simulink library "CPC5_SFUN_wrapper"  (Simulink 8.7)
settings: Solver=VariableStepAuto  SolverMode=SingleTasking  StartTime=0.0  StopTime=10.0  RelTol=1e-3
PreLoadFcn:
  | CPC5_SFUN_PreLoadFcn
  | CPC5_SFUN_InitFcn
undefined symbols (not defined in the file): user_config
settings Model: Creator=Silver T-2022.03-4  LastModifiedBy=pjhaver

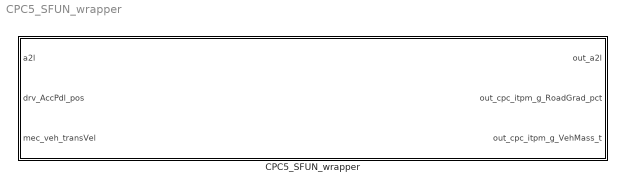
== system CPC5_SFUN_wrapper ==
  CPC5_SFUN_wrapper : Subsystem
      mask Display:
      | patch(.5 + 0.03*8*cos(0:pi/50:2*pi),   .5 + 0.14675 *8*sin(0:pi/50:2*pi), [0 0 1])
      | patch(.5 + 0.03*[6.5, 8, 0, -1.5],     .5 + 0.14675 *[-8,-6.5, 1.5, 0], [.8, .8, .8])
      | patch(.5 + 0.03*5.5*cos(0:pi/50:2*pi), .5 + 0.14675 *5.5*sin(0:pi/50:2*pi), [.8, .8, .8])
      | patch(.5 + 0.03*3.5*cos(0:pi/50:2*pi), .5 + 0.14675 *3.5*sin(0:pi/50:2*pi), [0 0 1])

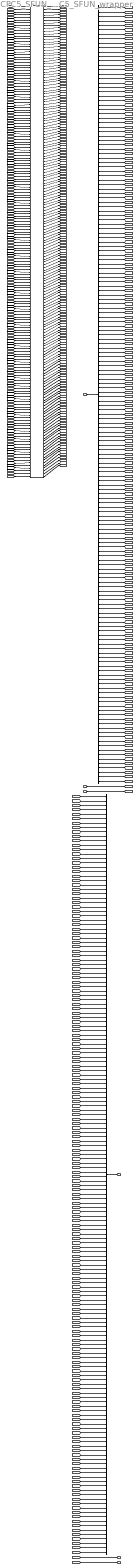
== system CPC5_SFUN_wrapper/CPC5_SFUN_wrapper ==
  a2l : Inport  OutDataTypeStr=Bus:a2l_1
  drv_AccPdl_pos : Inport  Port=2
  mec_veh_transVel : Inport  Port=3
  BusCreator183 : BusCreator  Inputs=172
  BusSelector1 : BusSelector  OutputSignals=ch_Accel_X_Cval,ch_AirTempOutsd_Cval_SCA,ch_AutoManSw_Rq_SAM,ch_BS_Brk_Cval,ch_BS_CSCPC_Acc_Stat,ch_BS_CSCPC_Intf_Stat,ch_BS_CSCPC_RqPerf_Stat,ch_BS_HB_RqPerf_Stat,ch_BrkPdlPosn3_Cval,ch_CC_DecHystSw_Rq,ch_CC_DecLoHystSw_Rq,ch_CC_HystSpd_Rq_ICUC,ch_CC_IncHystSw_Rq,ch_CC_IncLoHystSw_Rq,ch_CC_LowHystSpd_Rq_ICUC,ch_CstValIPPC_Rq,ch_CurvSpd_Rq,ch_DateTmDay_Cval_ICUC,ch_DateTmHour_Cval_ICUC,ch_DateTmMinute_Cval_ICUC,ch_DateTmMonth_Cval_ICUC,ch_DateTmSecond_Cval_ICUC,ch_DateTmYear_Cval_ICUC,ch_DiffLkIAC_Stat,ch_DipHystSpd_Rq,ch_DrvMdSwNorm_Rq_SAM,ch_EBS_BrkSw2_Rq,ch_EngRetTrqMax_Rq,ch_EngRetTrqMin_Rq,ch_GrSelSw_Rq_SAM,ch_HillHolderAvl_Stat,ch_IgnSw_Stat_SCA,ch_RetSwPos_Rq_SAM,ch_RoadCurv_Cval,ch_SFA_Ind_Stat,ch_SelSpdUnit_Stat,ch_SpdFtAxleLtWhl_Cval,ch_SpdFtAxleRtWhl_Cval,ch_SpdR_AxleLtWhl_Cval,ch_SpdR_AxleRtWhl_Cval,ch_SrcAdrBrkCtrlDev_Cval,ch_StW_Sw09_Rq,ch_StW_Sw10_Rq,ch_StW_Sw11_Rq,ch_StW_Sw13_Rq,ch_TotalVehDist_Cval_DIAG,ch_TrfGrBoxRng_Stat,ch_TyreRollCircumFA_Cval,ch_TyreRollCircumRA_Cval,ch_VehMtnDet_Stat_ICUC,ch_XBR_AccelLim_Stat_BS,pt_AbsMaxEngTrq_Cval_PT,pt_AbsMaxRetTrq_Cval_PT,pt_ActlMaxEngSpd_Cval_PT,pt_ActlMaxRetTrqNoTemp_Cval,pt_BoostPress_Cval_PT,pt_CC_MdDem_Rq,pt_Clutch_Cval_PT,pt_Clutch_Stat_TCM_PT,pt_CoolTempIn_Cval_PT,pt_CoolTempOut_Cval_PT,pt_CoolTempRet_Cval_PT,pt_CoolTemp_Cval_PT,pt_CreepAct_Stat_PT,pt_CreepMaxTrq_Cval_PT,pt_CurrGr_Stat_PT,pt_DeclSens_Cval_PT,pt_DrvDirByGr_Stat_TCM_PT,pt_DrvDirec_Stat_TCM_PT,pt_DrvlineEngg_Stat_PT,pt_EbmReq_IPPC,pt_EcoMode_Rq_PPC,pt_EngBrk1_Stat_MR_PT,pt_EngBrk2_Stat_MR_PT,pt_EngFrictTrq_Cval_PT,pt_EngHours_Cval_PT,pt_EngIdleSpd_Cval_MCM_PT,pt_EngIdleSpd_Rq_TCM_PT,pt_EngIdle_Stat_MCM,pt_EngIgn_Stat_MCM,pt_EngMode_Stat_MCM,pt_EngSpd_Cval_PT,pt_EngSpd_Rq_TCM_PT,pt_EngStSpInhbt_Rq_MCM,pt_EngTrqDecRate_Cval_PT,pt_EngTrq_Cval_PT,pt_FEL_Rq_IPPC,pt_FanSpdPct_Cval_PT,pt_FanSpd_Cval_PT,pt_FuelCons_Cval_PT,pt_FuelMapEngSpd_Cval_PT,pt_FuelMapNum_Cval_PT,pt_FuelMapSelNum_Cval_PT,pt_FuelMapTrqNoBst_Cval_PT,pt_FwdGr10_Stat_PT,pt_FwdGr11_Stat_PT,pt_FwdGr12_Stat_PT,pt_FwdGr13_Stat_PT,pt_FwdGr14_Stat_PT,pt_FwdGr15_Stat_PT,pt_FwdGr16_Stat_PT,pt_FwdGr1_Stat_PT,pt_FwdGr2_Stat_PT,pt_FwdGr3_Stat_PT,pt_FwdGr4_Stat_PT,pt_FwdGr5_Stat_PT,pt_FwdGr6_Stat_PT,pt_FwdGr7_Stat_PT,pt_FwdGr8_Stat_PT,pt_FwdGr9_Stat_PT,pt_GrShift_Stat_PT,pt_HystSpd_Cval_IPPC,pt_IPPC_Stat,pt_InShaftSpd_Cval_PT,pt_IntrUrbUcReq_IPPC,pt_LoHystSpd_Cval_IPPC,pt_LowSpd_Cval_IPPC,pt_MapRoadGrad_Cval,pt_MaxAccel_Rq_IPPC,pt_MaxActlEngTrq_Cval_PT,pt_MaxEngBrk_Rq_IPPC,pt_MaxEngTrq_Rq_PT,pt_MaxRetTrq_Cval_PT,pt_MinAccel_Rq_IPPC,pt_MinEngBrk_Rq_IPPC,pt_MinEngTrq_Rq_PT,pt_MinRetTrqPwrUp_Stat_PT,pt_NeuRangeGroup_Stat_PT,pt_NeuRangeHigh_Stat_PT,pt_NeuRangeLow_Stat_PT,pt_NeuSplitGroup_Stat_PT,pt_NeuSplitHigh_Stat_PT,pt_NeuSplitLow_Stat_PT,pt_OutShaftSpd_Cval_PT,pt_PThM_Blind_Rq_PT,pt_PThM_FanCtrl_Rq,pt_PThM_WtrPmp_Rq_PT,pt_PthM_ThstHeat_Rq_PT,pt_ReqTrq_Cval_IPPC,pt_RetActv_Stat_PT,pt_RetOilTemp_Cval_PT,pt_RetTrqMd_Stat,pt_RetTrq_Cval_PT,pt_RevGr2_Stat_PT,pt_RevGr3_Stat_PT,pt_RevGr4_Stat_PT,pt_RotSens_Stat_PT,pt_SOC_Range_Rq_IPPC,pt_SaveSetSpd_Rq_IPPC,pt_SelGr_Rq_IPPC,pt_SelGr_Stat_PT,pt_SelSpdController_Rq_PT,pt_SetSpd_Cval_IPPC,pt_ShiftSprtEng_Rq_TCM,pt_ShiftTimeDown1_Cval_PT,pt_ShiftTimeDown2_Cval_PT,pt_ShiftTimeDown3_Cval_PT,pt_ShiftTimeDown4_Cval_PT,pt_ShiftTimeUp1_Cval_PT,pt_ShiftTimeUp2_Cval_PT,pt_ShiftTimeUp3_Cval_PT,pt_ShiftTimeUp4_Cval_PT,pt_SysID_CCM,pt_SysID_MCM,pt_SysID_RCM,pt_SysID_TCM,pt_ThermoRoll_Rq,pt_TopTrq_Rq_IPPC,pt_TrqConvLkup_Stat_PT,pt_TrqConv_Cval_PT,pt_TrqConv_Stat_PT,pt_TxActlGrRatio_Cval_PT,pt_UpSpd_Cval_IPPC,pt_UseCase_Rq_IPPC,pt_XBR_Rq_IPPC,drv_ign
  sfunction : S-Function  FunctionName=CPC5_SFUN  Parameters=user_config  SFunctionDeploymentMode=off  EnableBusSupport=off  mask{user_config=user_config}
  out_a2l : Outport
  out_cpc_itpm_g_RoadGrad_pct : Outport  Port=2
  out_cpc_itpm_g_VehMass_t : Outport  Port=3
  wires:
  [L2] -> sfunction/1
  [L3] -> sfunction/2
  [L4] -> sfunction/3
  [L5] -> sfunction/4
  [L6] -> sfunction/5
  [L7] -> sfunction/6
  [L8] -> sfunction/7
  [L9] -> sfunction/8
  [L10] -> sfunction/9
  [L11] -> sfunction/10
  [L12] -> sfunction/11
  [L13] -> sfunction/12
  [L14] -> sfunction/13
  [L15] -> sfunction/14
  [L16] -> sfunction/15
  [L17] -> sfunction/16
  [L18] -> sfunction/17
  [L19] -> sfunction/18
  [L20] -> sfunction/19
  [L21] -> sfunction/20
  [L22] -> sfunction/21
  [L23] -> sfunction/22
  [L24] -> sfunction/23
  [L25] -> sfunction/24
  [L26] -> sfunction/25
  [L27] -> sfunction/26
  [L28] -> sfunction/27
  [L29] -> sfunction/28
  [L30] -> sfunction/29
  [L31] -> sfunction/30
  [L32] -> sfunction/31
  [L33] -> sfunction/32
  [L34] -> sfunction/33
  [L35] -> sfunction/34
  [L36] -> sfunction/35
  [L37] -> sfunction/36
  [L38] -> sfunction/37
  [L39] -> sfunction/38
  [L40] -> sfunction/39
  [L41] -> sfunction/40
  [L42] -> sfunction/41
  [L43] -> sfunction/42
  [L44] -> sfunction/43
  [L45] -> sfunction/44
  [L46] -> sfunction/45
  [L47] -> sfunction/46
  [L48] -> sfunction/47
  [L49] -> sfunction/48
  [L50] -> sfunction/49
  [L51] -> sfunction/50
  [L52] -> sfunction/51
  [L53] -> sfunction/52
  [L54] -> sfunction/53
  [L55] -> sfunction/54
  [L56] -> sfunction/55
  [L57] -> sfunction/56
  [L58] -> sfunction/57
  [L59] -> sfunction/58
  [L60] -> sfunction/59
  [L61] -> sfunction/60
  [L62] -> sfunction/61
  [L63] -> sfunction/62
  [L64] -> sfunction/63
  [L65] -> sfunction/64
  [L66] -> sfunction/65
  [L67] -> sfunction/66
  [L68] -> sfunction/67
  [L69] -> sfunction/68
  [L70] -> sfunction/69
  [L71] -> sfunction/70
  [L72] -> sfunction/71
  [L73] -> sfunction/72
  [L74] -> sfunction/73
  [L75] -> sfunction/74
  [L76] -> sfunction/75
  [L77] -> sfunction/76
  [L78] -> sfunction/77
  [L79] -> sfunction/78
  [L80] -> sfunction/79
  [L81] -> sfunction/80
  [L82] -> sfunction/81
  [L83] -> sfunction/82
  [L84] -> sfunction/83
  [L85] -> sfunction/84
  [L86] -> sfunction/85
  [L87] -> sfunction/86
  [L88] -> sfunction/87
  [L89] -> sfunction/88
  [L90] -> sfunction/89
  [L91] -> sfunction/90
  [L92] -> sfunction/91
  [L93] -> sfunction/92
  [L94] -> sfunction/93
  [L95] -> sfunction/94
  [L96] -> sfunction/95
  [L97] -> sfunction/96
  [L98] -> sfunction/97
  [L99] -> sfunction/98
  [L100] -> sfunction/99
  [L101] -> sfunction/100
  [L102] -> sfunction/101
  [L103] -> sfunction/102
  [L104] -> sfunction/103
  [L105] -> sfunction/104
  [L106] -> sfunction/105
  [L107] -> sfunction/106
  [L108] -> sfunction/107
  [L109] -> sfunction/108
  [L110] -> sfunction/109
  [L111] -> sfunction/110
  [L112] -> sfunction/111
  [L113] -> sfunction/112
  [L114] -> sfunction/113
  [L115] -> sfunction/114
  [L116] -> sfunction/115
  [L117] -> sfunction/116
  [L118] -> sfunction/117
  [L119] -> sfunction/118
  [L120] -> sfunction/119
  [L121] -> sfunction/120
  [L122] -> sfunction/121
  [L123] -> sfunction/122
  [L124] -> sfunction/123
  [L125] -> sfunction/124
  [L126] -> sfunction/125
  [L127] -> sfunction/126
  [L128] -> sfunction/127
  [L129] -> sfunction/128
  [L130] -> sfunction/129
  [L131] -> sfunction/130
  [L132] -> sfunction/131
  [L133] -> sfunction/132
  [L134] -> sfunction/133
  [L135] -> sfunction/134
  [L136] -> sfunction/135
  [L137] -> sfunction/136
  [L138] -> sfunction/137
  [L139] -> sfunction/138
  [L140] -> sfunction/139
  [L141] -> sfunction/140
  [L142] -> sfunction/141
  [L143] -> sfunction/142
  [L144] -> sfunction/143
  [L145] -> sfunction/144
  [L146] -> sfunction/145
  [L147] -> sfunction/146
  [L148] -> sfunction/147
  [L149] -> sfunction/148
  [L150] -> sfunction/149
  [L151] -> sfunction/150
  [L152] -> sfunction/151
  [L153] -> sfunction/152
  [L154] -> sfunction/153
  [L155] -> sfunction/154
  [L156] -> sfunction/155
  [L157] -> sfunction/156
  [L158] -> sfunction/157
  [L159] -> sfunction/158
  [L160] -> sfunction/159
  [L161] -> sfunction/160
  [L162] -> sfunction/161
  [L163] -> sfunction/162
  [L164] -> sfunction/163
  [L165] -> sfunction/164
  [L166] -> sfunction/165
  [L167] -> sfunction/166
  [L168] -> sfunction/167
  [L169] -> sfunction/168
  [L170] -> sfunction/169
  [L171] -> sfunction/170
  [L172] -> sfunction/171
  [L173] -> sfunction/172
  [L174] -> sfunction/173
  [L175] -> sfunction/174
  [L176] -> sfunction/175
  [L177] -> sfunction/177
  a2l/1 -> BusSelector1/1
  BusSelector1/1 -> [L2]  "<ch_Accel_X_Cval>"
  BusSelector1/2 -> [L3]  "<ch_AirTempOutsd_Cval_SCA>"
  BusSelector1/3 -> [L4]  "<ch_AutoManSw_Rq_SAM>"
  BusSelector1/4 -> [L5]  "<ch_BS_Brk_Cval>"
  BusSelector1/5 -> [L6]  "<ch_BS_CSCPC_Acc_Stat>"
  BusSelector1/6 -> [L7]  "<ch_BS_CSCPC_Intf_Stat>"
  BusSelector1/7 -> [L8]  "<ch_BS_CSCPC_RqPerf_Stat>"
  BusSelector1/8 -> [L9]  "<ch_BS_HB_RqPerf_Stat>"
  BusSelector1/9 -> [L10]  "<ch_BrkPdlPosn3_Cval>"
  BusSelector1/10 -> [L11]  "<ch_CC_DecHystSw_Rq>"
  BusSelector1/11 -> [L12]  "<ch_CC_DecLoHystSw_Rq>"
  BusSelector1/12 -> [L13]  "<ch_CC_HystSpd_Rq_ICUC>"
  BusSelector1/13 -> [L14]  "<ch_CC_IncHystSw_Rq>"
  BusSelector1/14 -> [L15]  "<ch_CC_IncLoHystSw_Rq>"
  BusSelector1/15 -> [L16]  "<ch_CC_LowHystSpd_Rq_ICUC>"
  BusSelector1/16 -> [L17]  "<ch_CstValIPPC_Rq>"
  BusSelector1/17 -> [L18]  "<ch_CurvSpd_Rq>"
  BusSelector1/18 -> [L19]  "<ch_DateTmDay_Cval_ICUC>"
  BusSelector1/19 -> [L20]  "<ch_DateTmHour_Cval_ICUC>"
  BusSelector1/20 -> [L21]  "<ch_DateTmMinute_Cval_ICUC>"
  BusSelector1/21 -> [L22]  "<ch_DateTmMonth_Cval_ICUC>"
  BusSelector1/22 -> [L23]  "<ch_DateTmSecond_Cval_ICUC>"
  BusSelector1/23 -> [L24]  "<ch_DateTmYear_Cval_ICUC>"
  BusSelector1/24 -> [L25]  "<ch_DiffLkIAC_Stat>"
  BusSelector1/25 -> [L26]  "<ch_DipHystSpd_Rq>"
  BusSelector1/26 -> [L27]  "<ch_DrvMdSwNorm_Rq_SAM>"
  BusSelector1/27 -> [L28]  "<ch_EBS_BrkSw2_Rq>"
  BusSelector1/28 -> [L29]  "<ch_EngRetTrqMax_Rq>"
  BusSelector1/29 -> [L30]  "<ch_EngRetTrqMin_Rq>"
  BusSelector1/30 -> [L31]  "<ch_GrSelSw_Rq_SAM>"
  BusSelector1/31 -> [L32]  "<ch_HillHolderAvl_Stat>"
  BusSelector1/32 -> [L33]  "<ch_IgnSw_Stat_SCA>"
  BusSelector1/33 -> [L34]  "<ch_RetSwPos_Rq_SAM>"
  BusSelector1/34 -> [L35]  "<ch_RoadCurv_Cval>"
  BusSelector1/35 -> [L36]  "<ch_SFA_Ind_Stat>"
  BusSelector1/36 -> [L37]  "<ch_SelSpdUnit_Stat>"
  BusSelector1/37 -> [L38]  "<ch_SpdFtAxleLtWhl_Cval>"
  BusSelector1/38 -> [L39]  "<ch_SpdFtAxleRtWhl_Cval>"
  BusSelector1/39 -> [L40]  "<ch_SpdR_AxleLtWhl_Cval>"
  BusSelector1/40 -> [L41]  "<ch_SpdR_AxleRtWhl_Cval>"
  BusSelector1/41 -> [L42]  "<ch_SrcAdrBrkCtrlDev_Cval>"
  BusSelector1/42 -> [L43]  "<ch_StW_Sw09_Rq>"
  BusSelector1/43 -> [L44]  "<ch_StW_Sw10_Rq>"
  BusSelector1/44 -> [L45]  "<ch_StW_Sw11_Rq>"
  BusSelector1/45 -> [L46]  "<ch_StW_Sw13_Rq>"
  BusSelector1/46 -> [L47]  "<ch_TotalVehDist_Cval_DIAG>"
  BusSelector1/47 -> [L48]  "<ch_TrfGrBoxRng_Stat>"
  BusSelector1/48 -> [L49]  "<ch_TyreRollCircumFA_Cval>"
  BusSelector1/49 -> [L50]  "<ch_TyreRollCircumRA_Cval>"
  BusSelector1/50 -> [L51]  "<ch_VehMtnDet_Stat_ICUC>"
  BusSelector1/51 -> [L52]  "<ch_XBR_AccelLim_Stat_BS>"
  BusSelector1/52 -> [L53]  "<pt_AbsMaxEngTrq_Cval_PT>"
  BusSelector1/53 -> [L54]  "<pt_AbsMaxRetTrq_Cval_PT>"
  BusSelector1/54 -> [L55]  "<pt_ActlMaxEngSpd_Cval_PT>"
  BusSelector1/55 -> [L56]  "<pt_ActlMaxRetTrqNoTemp_Cval>"
  BusSelector1/56 -> [L57]  "<pt_BoostPress_Cval_PT>"
  BusSelector1/57 -> [L58]  "<pt_CC_MdDem_Rq>"
  BusSelector1/58 -> [L59]  "<pt_Clutch_Cval_PT>"
  BusSelector1/59 -> [L60]  "<pt_Clutch_Stat_TCM_PT>"
  BusSelector1/60 -> [L61]  "<pt_CoolTempIn_Cval_PT>"
  BusSelector1/61 -> [L62]  "<pt_CoolTempOut_Cval_PT>"
  BusSelector1/62 -> [L63]  "<pt_CoolTempRet_Cval_PT>"
  BusSelector1/63 -> [L64]  "<pt_CoolTemp_Cval_PT>"
  BusSelector1/64 -> [L65]  "<pt_CreepAct_Stat_PT>"
  BusSelector1/65 -> [L66]  "<pt_CreepMaxTrq_Cval_PT>"
  BusSelector1/66 -> [L67]  "<pt_CurrGr_Stat_PT>"
  BusSelector1/67 -> [L68]  "<pt_DeclSens_Cval_PT>"
  BusSelector1/68 -> [L69]  "<pt_DrvDirByGr_Stat_TCM_PT>"
  BusSelector1/69 -> [L70]  "<pt_DrvDirec_Stat_TCM_PT>"
  BusSelector1/70 -> [L71]  "<pt_DrvlineEngg_Stat_PT>"
  BusSelector1/71 -> [L72]  "<pt_EbmReq_IPPC>"
  BusSelector1/72 -> [L73]  "<pt_EcoMode_Rq_PPC>"
  BusSelector1/73 -> [L74]  "<pt_EngBrk1_Stat_MR_PT>"
  BusSelector1/74 -> [L75]  "<pt_EngBrk2_Stat_MR_PT>"
  BusSelector1/75 -> [L76]  "<pt_EngFrictTrq_Cval_PT>"
  BusSelector1/76 -> [L77]  "<pt_EngHours_Cval_PT>"
  BusSelector1/77 -> [L78]  "<pt_EngIdleSpd_Cval_MCM_PT>"
  BusSelector1/78 -> [L79]  "<pt_EngIdleSpd_Rq_TCM_PT>"
  BusSelector1/79 -> [L80]  "<pt_EngIdle_Stat_MCM>"
  BusSelector1/80 -> [L81]  "<pt_EngIgn_Stat_MCM>"
  BusSelector1/81 -> [L82]  "<pt_EngMode_Stat_MCM>"
  BusSelector1/82 -> [L83]  "<pt_EngSpd_Cval_PT>"
  BusSelector1/83 -> [L84]  "<pt_EngSpd_Rq_TCM_PT>"
  BusSelector1/84 -> [L85]  "<pt_EngStSpInhbt_Rq_MCM>"
  BusSelector1/85 -> [L86]  "<pt_EngTrqDecRate_Cval_PT>"
  BusSelector1/86 -> [L87]  "<pt_EngTrq_Cval_PT>"
  BusSelector1/87 -> [L88]  "<pt_FEL_Rq_IPPC>"
  BusSelector1/88 -> [L89]  "<pt_FanSpdPct_Cval_PT>"
  BusSelector1/89 -> [L90]  "<pt_FanSpd_Cval_PT>"
  BusSelector1/90 -> [L91]  "<pt_FuelCons_Cval_PT>"
  BusSelector1/91 -> [L92]  "<pt_FuelMapEngSpd_Cval_PT>"
  BusSelector1/92 -> [L93]  "<pt_FuelMapNum_Cval_PT>"
  BusSelector1/93 -> [L94]  "<pt_FuelMapSelNum_Cval_PT>"
  BusSelector1/94 -> [L95]  "<pt_FuelMapTrqNoBst_Cval_PT>"
  BusSelector1/95 -> [L96]  "<pt_FwdGr10_Stat_PT>"
  BusSelector1/96 -> [L97]  "<pt_FwdGr11_Stat_PT>"
  BusSelector1/97 -> [L98]  "<pt_FwdGr12_Stat_PT>"
  BusSelector1/98 -> [L99]  "<pt_FwdGr13_Stat_PT>"
  BusSelector1/99 -> [L100]  "<pt_FwdGr14_Stat_PT>"
  BusSelector1/100 -> [L101]  "<pt_FwdGr15_Stat_PT>"
  BusSelector1/101 -> [L102]  "<pt_FwdGr16_Stat_PT>"
  BusSelector1/102 -> [L103]  "<pt_FwdGr1_Stat_PT>"
  BusSelector1/103 -> [L104]  "<pt_FwdGr2_Stat_PT>"
  BusSelector1/104 -> [L105]  "<pt_FwdGr3_Stat_PT>"
  BusSelector1/105 -> [L106]  "<pt_FwdGr4_Stat_PT>"
  BusSelector1/106 -> [L107]  "<pt_FwdGr5_Stat_PT>"
  BusSelector1/107 -> [L108]  "<pt_FwdGr6_Stat_PT>"
  BusSelector1/108 -> [L109]  "<pt_FwdGr7_Stat_PT>"
  BusSelector1/109 -> [L110]  "<pt_FwdGr8_Stat_PT>"
  BusSelector1/110 -> [L111]  "<pt_FwdGr9_Stat_PT>"
  BusSelector1/111 -> [L112]  "<pt_GrShift_Stat_PT>"
  BusSelector1/112 -> [L113]  "<pt_HystSpd_Cval_IPPC>"
  BusSelector1/113 -> [L114]  "<pt_IPPC_Stat>"
  BusSelector1/114 -> [L115]  "<pt_InShaftSpd_Cval_PT>"
  BusSelector1/115 -> [L116]  "<pt_IntrUrbUcReq_IPPC>"
  BusSelector1/116 -> [L117]  "<pt_LoHystSpd_Cval_IPPC>"
  BusSelector1/117 -> [L118]  "<pt_LowSpd_Cval_IPPC>"
  BusSelector1/118 -> [L119]  "<pt_MapRoadGrad_Cval>"
  BusSelector1/119 -> [L120]  "<pt_MaxAccel_Rq_IPPC>"
  BusSelector1/120 -> [L121]  "<pt_MaxActlEngTrq_Cval_PT>"
  BusSelector1/121 -> [L122]  "<pt_MaxEngBrk_Rq_IPPC>"
  BusSelector1/122 -> [L123]  "<pt_MaxEngTrq_Rq_PT>"
  BusSelector1/123 -> [L124]  "<pt_MaxRetTrq_Cval_PT>"
  BusSelector1/124 -> [L125]  "<pt_MinAccel_Rq_IPPC>"
  BusSelector1/125 -> [L126]  "<pt_MinEngBrk_Rq_IPPC>"
  BusSelector1/126 -> [L127]  "<pt_MinEngTrq_Rq_PT>"
  BusSelector1/127 -> [L128]  "<pt_MinRetTrqPwrUp_Stat_PT>"
  BusSelector1/128 -> [L129]  "<pt_NeuRangeGroup_Stat_PT>"
  BusSelector1/129 -> [L130]  "<pt_NeuRangeHigh_Stat_PT>"
  BusSelector1/130 -> [L131]  "<pt_NeuRangeLow_Stat_PT>"
  BusSelector1/131 -> [L132]  "<pt_NeuSplitGroup_Stat_PT>"
  BusSelector1/132 -> [L133]  "<pt_NeuSplitHigh_Stat_PT>"
  BusSelector1/133 -> [L134]  "<pt_NeuSplitLow_Stat_PT>"
  BusSelector1/134 -> [L135]  "<pt_OutShaftSpd_Cval_PT>"
  BusSelector1/135 -> [L136]  "<pt_PThM_Blind_Rq_PT>"
  BusSelector1/136 -> [L137]  "<pt_PThM_FanCtrl_Rq>"
  BusSelector1/137 -> [L138]  "<pt_PThM_WtrPmp_Rq_PT>"
  BusSelector1/138 -> [L139]  "<pt_PthM_ThstHeat_Rq_PT>"
  BusSelector1/139 -> [L140]  "<pt_ReqTrq_Cval_IPPC>"
  BusSelector1/140 -> [L141]  "<pt_RetActv_Stat_PT>"
  BusSelector1/141 -> [L142]  "<pt_RetOilTemp_Cval_PT>"
  BusSelector1/142 -> [L143]  "<pt_RetTrqMd_Stat>"
  BusSelector1/143 -> [L144]  "<pt_RetTrq_Cval_PT>"
  BusSelector1/144 -> [L145]  "<pt_RevGr2_Stat_PT>"
  BusSelector1/145 -> [L146]  "<pt_RevGr3_Stat_PT>"
  BusSelector1/146 -> [L147]  "<pt_RevGr4_Stat_PT>"
  BusSelector1/147 -> [L148]  "<pt_RotSens_Stat_PT>"
  BusSelector1/148 -> [L149]  "<pt_SOC_Range_Rq_IPPC>"
  BusSelector1/149 -> [L150]  "<pt_SaveSetSpd_Rq_IPPC>"
  BusSelector1/150 -> [L151]  "<pt_SelGr_Rq_IPPC>"
  BusSelector1/151 -> [L152]  "<pt_SelGr_Stat_PT>"
  BusSelector1/152 -> [L153]  "<pt_SelSpdController_Rq_PT>"
  BusSelector1/153 -> [L154]  "<pt_SetSpd_Cval_IPPC>"
  BusSelector1/154 -> [L155]  "<pt_ShiftSprtEng_Rq_TCM>"
  BusSelector1/155 -> [L156]  "<pt_ShiftTimeDown1_Cval_PT>"
  BusSelector1/156 -> [L157]  "<pt_ShiftTimeDown2_Cval_PT>"
  BusSelector1/157 -> [L158]  "<pt_ShiftTimeDown3_Cval_PT>"
  BusSelector1/158 -> [L159]  "<pt_ShiftTimeDown4_Cval_PT>"
  BusSelector1/159 -> [L160]  "<pt_ShiftTimeUp1_Cval_PT>"
  BusSelector1/160 -> [L161]  "<pt_ShiftTimeUp2_Cval_PT>"
  BusSelector1/161 -> [L162]  "<pt_ShiftTimeUp3_Cval_PT>"
  BusSelector1/162 -> [L163]  "<pt_ShiftTimeUp4_Cval_PT>"
  BusSelector1/163 -> [L164]  "<pt_SysID_CCM>"
  BusSelector1/164 -> [L165]  "<pt_SysID_MCM>"
  BusSelector1/165 -> [L166]  "<pt_SysID_RCM>"
  BusSelector1/166 -> [L167]  "<pt_SysID_TCM>"
  BusSelector1/167 -> [L168]  "<pt_ThermoRoll_Rq>"
  BusSelector1/168 -> [L169]  "<pt_TopTrq_Rq_IPPC>"
  BusSelector1/169 -> [L170]  "<pt_TrqConvLkup_Stat_PT>"
  BusSelector1/170 -> [L171]  "<pt_TrqConv_Cval_PT>"
  BusSelector1/171 -> [L172]  "<pt_TrqConv_Stat_PT>"
  BusSelector1/172 -> [L173]  "<pt_TxActlGrRatio_Cval_PT>"
  BusSelector1/173 -> [L174]  "<pt_UpSpd_Cval_IPPC>"
  BusSelector1/174 -> [L175]  "<pt_UseCase_Rq_IPPC>"
  BusSelector1/175 -> [L176]  "<pt_XBR_Rq_IPPC>"
  BusSelector1/176 -> [L177]  "<drv_ign>"
  drv_AccPdl_pos/1 -> [L179]
  [L179] -> sfunction/176
  mec_veh_transVel/1 -> [L180]
  [L180] -> sfunction/178
  sfunction/1 -> [L184]
  sfunction/2 -> [L185]
  sfunction/3 -> [L186]
  sfunction/4 -> [L187]
  sfunction/5 -> [L188]
  sfunction/6 -> [L189]
  sfunction/7 -> [L190]
  sfunction/8 -> [L191]
  sfunction/9 -> [L192]
  sfunction/10 -> [L193]
  sfunction/11 -> [L194]
  sfunction/12 -> [L195]
  sfunction/13 -> [L196]
  sfunction/14 -> [L197]
  sfunction/15 -> [L198]
  sfunction/16 -> [L199]
  sfunction/17 -> [L200]
  sfunction/18 -> [L201]
  sfunction/19 -> [L202]
  sfunction/20 -> [L203]
  sfunction/21 -> [L204]
  sfunction/22 -> [L205]
  sfunction/23 -> [L206]
  sfunction/24 -> [L207]
  sfunction/25 -> [L208]
  sfunction/26 -> [L209]
  sfunction/27 -> [L210]
  sfunction/28 -> [L211]
  sfunction/29 -> [L212]
  sfunction/30 -> [L213]
  sfunction/31 -> [L214]
  sfunction/32 -> [L215]
  sfunction/33 -> [L216]
  sfunction/34 -> [L217]
  sfunction/35 -> [L218]
  sfunction/36 -> [L219]
  sfunction/37 -> [L220]
  sfunction/38 -> [L221]
  sfunction/39 -> [L222]
  sfunction/40 -> [L223]
  sfunction/41 -> [L224]
  sfunction/42 -> [L225]
  sfunction/43 -> [L226]
  sfunction/44 -> [L227]
  sfunction/45 -> [L228]
  sfunction/46 -> [L229]
  sfunction/47 -> [L230]
  sfunction/48 -> [L231]
  sfunction/49 -> [L232]
  sfunction/50 -> [L233]
  sfunction/51 -> [L234]
  sfunction/52 -> [L235]
  sfunction/53 -> [L236]
  sfunction/54 -> [L237]
  sfunction/55 -> [L238]
  sfunction/56 -> [L239]
  sfunction/57 -> [L240]
  sfunction/58 -> [L241]
  sfunction/59 -> [L242]
  sfunction/60 -> [L243]
  sfunction/61 -> [L244]
  sfunction/62 -> [L245]
  sfunction/63 -> [L246]
  sfunction/64 -> [L247]
  sfunction/65 -> [L248]
  sfunction/66 -> [L249]
  sfunction/67 -> [L250]
  sfunction/68 -> [L251]
  sfunction/69 -> [L252]
  sfunction/70 -> [L253]
  sfunction/71 -> [L254]
  sfunction/72 -> [L255]
  sfunction/73 -> [L256]
  sfunction/74 -> [L257]
  sfunction/75 -> [L258]
  sfunction/76 -> [L259]
  sfunction/77 -> [L260]
  sfunction/78 -> [L261]
  sfunction/79 -> [L262]
  sfunction/80 -> [L263]
  sfunction/81 -> [L264]
  sfunction/82 -> [L265]
  sfunction/83 -> [L266]
  sfunction/84 -> [L267]
  sfunction/85 -> [L268]
  sfunction/86 -> [L269]
  sfunction/87 -> [L270]
  sfunction/88 -> [L271]
  sfunction/89 -> [L272]
  sfunction/90 -> [L273]
  sfunction/91 -> [L274]
  sfunction/92 -> [L275]
  sfunction/93 -> [L276]
  sfunction/94 -> [L277]
  sfunction/95 -> [L278]
  sfunction/96 -> [L279]
  sfunction/97 -> [L280]
  sfunction/98 -> [L281]
  sfunction/99 -> [L282]
  sfunction/100 -> [L283]
  sfunction/101 -> [L284]
  sfunction/102 -> [L285]
  sfunction/103 -> [L286]
  sfunction/104 -> [L287]
  sfunction/105 -> [L288]
  sfunction/106 -> [L289]
  sfunction/107 -> [L290]
  sfunction/108 -> [L291]
  sfunction/109 -> [L292]
  sfunction/110 -> [L293]
  sfunction/111 -> [L294]
  sfunction/112 -> [L295]
  sfunction/113 -> [L296]
  sfunction/114 -> [L297]
  sfunction/115 -> [L298]
  sfunction/116 -> [L299]
  sfunction/117 -> [L300]
  sfunction/118 -> [L301]
  sfunction/119 -> [L302]
  sfunction/120 -> [L303]
  sfunction/121 -> [L304]
  sfunction/122 -> [L305]
  sfunction/123 -> [L306]
  sfunction/124 -> [L307]
  sfunction/125 -> [L308]
  sfunction/126 -> [L309]
  sfunction/127 -> [L310]
  sfunction/128 -> [L311]
  sfunction/129 -> [L312]
  sfunction/130 -> [L313]
  sfunction/131 -> [L314]
  sfunction/132 -> [L315]
  sfunction/133 -> [L316]
  sfunction/134 -> [L317]
  sfunction/135 -> [L318]
  sfunction/136 -> [L319]
  sfunction/137 -> [L320]
  sfunction/138 -> [L321]
  sfunction/139 -> [L322]
  sfunction/140 -> [L323]
  sfunction/141 -> [L324]
  sfunction/142 -> [L325]
  sfunction/143 -> [L326]
  sfunction/144 -> [L327]
  sfunction/145 -> [L328]
  sfunction/146 -> [L329]
  sfunction/147 -> [L330]
  sfunction/148 -> [L331]
  sfunction/149 -> [L332]
  sfunction/150 -> [L333]
  sfunction/151 -> [L334]
  sfunction/152 -> [L335]
  sfunction/153 -> [L336]
  sfunction/154 -> [L337]
  sfunction/155 -> [L338]
  sfunction/156 -> [L339]
  sfunction/157 -> [L340]
  sfunction/158 -> [L341]
  sfunction/159 -> [L342]
  sfunction/160 -> [L343]
  sfunction/161 -> [L344]
  sfunction/162 -> [L345]
  sfunction/163 -> [L346]
  sfunction/164 -> [L347]
  sfunction/165 -> [L348]
  sfunction/166 -> [L349]
  sfunction/167 -> [L350]
  sfunction/168 -> [L351]
  sfunction/169 -> [L352]
  sfunction/170 -> [L353]
  sfunction/171 -> [L354]
  sfunction/172 -> [L355]
  BusCreator183/1 -> out_a2l/1
  [L184] -> BusCreator183/1  "out_ch_AccelPdlLoIdleSw_Stat"
  [L185] -> BusCreator183/2  "out_ch_AccelPdlPosn_Cval"
  [L186] -> BusCreator183/3  "out_ch_ActOffCond_Stat"
  [L187] -> BusCreator183/4  "out_ch_ActlEmotTrq_Cval"
  [L188] -> BusCreator183/5  "out_ch_ActlEngPctTrq_Cval"
  [L189] -> BusCreator183/6  "out_ch_ActlMaxAvlRetPctTrq_Cval_CPC3"
  [L190] -> BusCreator183/7  "out_ch_ActlRetPctTrq_Cval_CPC3"
  [L191] -> BusCreator183/8  "out_ch_AutoSetSpdMd_Stat"
  [L192] -> BusCreator183/9  "out_ch_CC_Actv_Stat"
  [L193] -> BusCreator183/10  "out_ch_CC_Actvn_Stat"
  [L194] -> BusCreator183/11  "out_ch_CC_BrkSpd_Cval"
  [L195] -> BusCreator183/12  "out_ch_CC_FuncMode_Stat"
  [L196] -> BusCreator183/13  "out_ch_CC_HiResSetSpd_Cval"
  [L197] -> BusCreator183/14  "out_ch_CC_HystSpd_Cval"
  [L198] -> BusCreator183/15  "out_ch_CC_SetSpd_Cval"
  [L199] -> BusCreator183/16  "out_ch_Clutch_Stat_CPC"
  [L200] -> BusCreator183/17  "out_ch_DeclSens_Cval_PT"
  [L201] -> BusCreator183/18  "out_ch_DispAutoMan_Rq_CPC"
  [L202] -> BusCreator183/19  "out_ch_DispEngSp_Rq"
  [L203] -> BusCreator183/20  "out_ch_DispEngStSp_Stat"
  [L204] -> BusCreator183/21  "out_ch_DrvDirec2_Stat_CPC"
  [L205] -> BusCreator183/22  "out_ch_DrvDirec_Stat_TCM_PT"
  [L206] -> BusCreator183/23  "out_ch_EngPctTrqDrv_Rq"
  [L207] -> BusCreator183/24  "out_ch_EngRPM_Cval_CPC3"
  [L208] -> BusCreator183/25  "out_ch_EngRefTrq_Cval"
  [L209] -> BusCreator183/26  "out_ch_EngShutDownMSS_Stat"
  [L210] -> BusCreator183/27  "out_ch_EngStSp_Stat"
  [L211] -> BusCreator183/28  "out_ch_ExtAccel_Rq_CPC"
  [L212] -> BusCreator183/29  "out_ch_ExtBrkStat_Rq_CPC"
  [L213] -> BusCreator183/30  "out_ch_FanSpdPct_Cval_PT"
  [L214] -> BusCreator183/31  "out_ch_FanSpd_Cval_PT"
  [L215] -> BusCreator183/32  "out_ch_FuncLmpRET_Rq"
  [L216] -> BusCreator183/33  "out_ch_GrShift_Stat_PT"
  [L217] -> BusCreator183/34  "out_ch_HB_Rq_Stat_CPC"
  [L218] -> BusCreator183/35  "out_ch_LastGrRlsRsn_Stat"
  [L219] -> BusCreator183/36  "out_ch_MC_E3_Cval_CPC"
  [L220] -> BusCreator183/37  "out_ch_NomFrictEngPctTrq_Cval"
  [L221] -> BusCreator183/38  "out_ch_PtRt_Cval_CH"
  [L222] -> BusCreator183/39  "out_ch_RetPctTrqActl2_Cval_CPC3"
  [L223] -> BusCreator183/40  "out_ch_RetRefTrq_Cval"
  [L224] -> BusCreator183/41  "out_ch_RetSwPos_Rq_STSR"
  [L225] -> BusCreator183/42  "out_ch_RetTrqMd_Stat_CPC3"
  [L226] -> BusCreator183/43  "out_ch_RetTrq_Cval_PT"
  [L227] -> BusCreator183/44  "out_ch_SLDrvMdSw_Stat"
  [L228] -> BusCreator183/45  "out_ch_ShiftPrg_Stat"
  [L229] -> BusCreator183/46  "out_ch_SrvBrkSw_Stat"
  [L230] -> BusCreator183/47  "out_ch_TargetEngTrqCpc_Rq"
  [L231] -> BusCreator183/48  "out_ch_TrqConvLkup_Stat_PT"
  [L232] -> BusCreator183/49  "out_ch_TrqConv_Cval_PT"
  [L233] -> BusCreator183/50  "out_ch_TrqConv_Stat_PT"
  [L234] -> BusCreator183/51  "out_ch_TxActlGrRatio_Cval"
  [L235] -> BusCreator183/52  "out_ch_TxClutchPctSlp_Cval_CPC"
  [L236] -> BusCreator183/53  "out_ch_TxCurrGr_Stat"
  [L237] -> BusCreator183/54  "out_ch_TxDrvlineEngg_Stat_CPC"
  [L238] -> BusCreator183/55  "out_ch_TxInShaftSpd_Cval_CPC"
  [L239] -> BusCreator183/56  "out_ch_TxOutShaftSpd_Cval_CPC"
  [L240] -> BusCreator183/57  "out_ch_TxShftIP_Stat_CPC"
  [L241] -> BusCreator183/58  "out_ch_VehSpd_Cval_CPC"
  [L242] -> BusCreator183/59  "out_pt_ACC_CtrlDmnt_Stat"
  [L243] -> BusCreator183/60  "out_pt_ATC_Ctrl_Stat_PT"
  [L244] -> BusCreator183/61  "out_pt_AccelPdlKickDnSw_Rq"
  [L245] -> BusCreator183/62  "out_pt_AccelPdlLoIdleSw_Stat"
  [L246] -> BusCreator183/63  "out_pt_AccelPdlPosn_Cval"
  [L247] -> BusCreator183/64  "out_pt_AmbTemp_Cval_PT"
  [L248] -> BusCreator183/65  "out_pt_AutoSetSpdMd_Stat"
  [L249] -> BusCreator183/66  "out_pt_BS_Brk_Cval"
  [L250] -> BusCreator183/67  "out_pt_BrkPdlPosn3_Cval"
  [L251] -> BusCreator183/68  "out_pt_CC_Actvn_Stat_PT"
  [L252] -> BusCreator183/69  "out_pt_CC_FuncMode_Stat"
  [L253] -> BusCreator183/70  "out_pt_CC_HystSpd2_Cval"
  [L254] -> BusCreator183/71  "out_pt_CC_HystSpd_Cval"
  [L255] -> BusCreator183/72  "out_pt_CC_LoHystSpd2_Cval"
  [L256] -> BusCreator183/73  "out_pt_CC_LoHystSpd_Cval"
  [L257] -> BusCreator183/74  "out_pt_CC_Md_Stat"
  [L258] -> BusCreator183/75  "out_pt_CC_SaveSetSpd_Rs"
  [L259] -> BusCreator183/76  "out_pt_CC_SetSpd3_Cval"
  [L260] -> BusCreator183/77  "out_pt_CC_SetSpd_Cval"
  [L261] -> BusCreator183/78  "out_pt_CC_SetSpd_Estm_Cval"
  [L262] -> BusCreator183/79  "out_pt_CPC_IdleCond_Stat_PT"
  [L263] -> BusCreator183/80  "out_pt_ClutchCls_Stat_PT"
  [L264] -> BusCreator183/81  "out_pt_ClutchOpn_Rq_CPC"
  [L265] -> BusCreator183/82  "out_pt_ClutchOpn_Stat_PT"
  [L266] -> BusCreator183/83  "out_pt_CoolLvl_Stat_PT"
  [L267] -> BusCreator183/84  "out_pt_CstValIPPC_Stat"
  [L268] -> BusCreator183/85  "out_pt_CurrManGr_Stat_PT"
  [L269] -> BusCreator183/86  "out_pt_CurvSpd_Stat"
  [L270] -> BusCreator183/87  "out_pt_CutoffFreqSurgDamp_Cval_PT"
  [L271] -> BusCreator183/88  "out_pt_DPF_InhbtRegen_Rq_PT"
  [L272] -> BusCreator183/89  "out_pt_DateTmDay_Cval_ICUC"
  [L273] -> BusCreator183/90  "out_pt_DateTmHour_Cval_ICUC"
  [L274] -> BusCreator183/91  "out_pt_DateTmMinute_Cval_ICUC"
  [L275] -> BusCreator183/92  "out_pt_DateTmMonth_Cval_ICUC"
  [L276] -> BusCreator183/93  "out_pt_DateTmSecond_Cval_ICUC"
  [L277] -> BusCreator183/94  "out_pt_DateTmYear_Cval_ICUC"
  [L278] -> BusCreator183/95  "out_pt_DipHystSpd_Cval"
  [L279] -> BusCreator183/96  "out_pt_DisturbanceTrq_Cal"
  [L280] -> BusCreator183/97  "out_pt_DrvFriction_Cval_PT"
  [L281] -> BusCreator183/98  "out_pt_DynWhlRadius_Cval"
  [L282] -> BusCreator183/99  "out_pt_EcoRollMd_Stat"
  [L283] -> BusCreator183/100  "out_pt_EcoRollNeu_Rq_PT"
  [L284] -> BusCreator183/101  "out_pt_EngBrk1_Rq_PT"
  [L285] -> BusCreator183/102  "out_pt_EngBrk2_Rq_PT"
  [L286] -> BusCreator183/103  "out_pt_EngCrk_Stat"
  [L287] -> BusCreator183/104  "out_pt_EngExtStart_Stat_PT"
  [L288] -> BusCreator183/105  "out_pt_EngIdle_Stat_PT"
  [L289] -> BusCreator183/106  "out_pt_EngIgn_Stat_PT"
  [L290] -> BusCreator183/107  "out_pt_EngSpd_Rq_PT"
  [L291] -> BusCreator183/108  "out_pt_EngStrtr_Stat_PT"
  [L292] -> BusCreator183/109  "out_pt_EngTrq_Rq_PT"
  [L293] -> BusCreator183/110  "out_pt_EngZeroTrq_Stat_PT"
  [L294] -> BusCreator183/111  "out_pt_Fan_Rq_PT"
  [L295] -> BusCreator183/112  "out_pt_FuelLvl_Cval"
  [L296] -> BusCreator183/113  "out_pt_FuelMapSel_Rq_PT"
  [L297] -> BusCreator183/114  "out_pt_GaimSurgDamp_Cval_PT"
  [L298] -> BusCreator183/115  "out_pt_GovType_Stat_PT"
  [L299] -> BusCreator183/116  "out_pt_HiResAccelPdlPosn_Cval"
  [L300] -> BusCreator183/117  "out_pt_IPPC_Md2_Stat"
  [L301] -> BusCreator183/118  "out_pt_IPPC_Md_Rq"
  [L302] -> BusCreator183/119  "out_pt_IgnSw_Stat_SCA"
  [L303] -> BusCreator183/120  "out_pt_IntrUrbMd_Stat"
  [L304] -> BusCreator183/121  "out_pt_KickDn_Stat_PT"
  [L305] -> BusCreator183/122  "out_pt_LimGovDroopSpd_Cval"
  [L306] -> BusCreator183/123  "out_pt_LocalMinuteOffset_Cval_ICUC"
  [L307] -> BusCreator183/124  "out_pt_MaxEngSpd_Cval_PT"
  [L308] -> BusCreator183/125  "out_pt_MinEngSpd_Cval_PT"
  [L309] -> BusCreator183/126  "out_pt_MomntOver_Rq_PT"
  [L310] -> BusCreator183/127  "out_pt_NeuRangeGroup_Rq_PT"
  [L311] -> BusCreator183/128  "out_pt_NeuSplitGroup_Rq_PT"
  [L312] -> BusCreator183/129  "out_pt_NeuSw_Stat_PT"
  [L313] -> BusCreator183/130  "out_pt_ObsDrvFriction_Cval_PT"
  [L314] -> BusCreator183/131  "out_pt_ObsSel_Cval"
  [L315] -> BusCreator183/132  "out_pt_PTO_EstmTrq_Cval"
  [L316] -> BusCreator183/133  "out_pt_PrkBrk_Stat_PT"
  [L317] -> BusCreator183/134  "out_pt_RegenActv_Rq_CPC"
  [L318] -> BusCreator183/135  "out_pt_RetSwPosn2_Stat_PT"
  [L319] -> BusCreator183/136  "out_pt_RetTrq_Rq_PT"
  [L320] -> BusCreator183/137  "out_pt_RlsSelGr_Rq_PT"
  [L321] -> BusCreator183/138  "out_pt_RoadGrad_Cval_PT"
  [L322] -> BusCreator183/139  "out_pt_RoadGrad_Stat_PT"
  [L323] -> BusCreator183/140  "out_pt_SPEEDO_ZeSig_Stat_PT"
  [L324] -> BusCreator183/141  "out_pt_SelGr_Rq_PT"
  [L325] -> BusCreator183/142  "out_pt_ShiftMd_Stat"
  [L326] -> BusCreator183/143  "out_pt_ShiftPrg_Stat"
  [L327] -> BusCreator183/144  "out_pt_ShiftSprtEng_Rq_PT"
  [L328] -> BusCreator183/145  "out_pt_SpdFtAxleLtWhl_Cval"
  [L329] -> BusCreator183/146  "out_pt_SpdFtAxleRtWhl_Cval"
  [L330] -> BusCreator183/147  "out_pt_SpdR_AxleLtWhl_Cval"
  [L331] -> BusCreator183/148  "out_pt_SpdR_AxleRtWhl_Cval"
  [L332] -> BusCreator183/149  "out_pt_SrvBrkSw_Stat_PT"
  [L333] -> BusCreator183/150  "out_pt_SurgeDamp_Stat_PT"
  [L334] -> BusCreator183/151  "out_pt_SysID_CPC3"
  [L335] -> BusCreator183/152  "out_pt_TargetEngTrqETP_Rq_PT"
  [L336] -> BusCreator183/153  "out_pt_TargetEngTrqRQV_Rq_PT"
  [L337] -> BusCreator183/154  "out_pt_TargetEngTrq_Rq_PT"
  [L338] -> BusCreator183/155  "out_pt_ThermoHt_Rq_PT"
  [L339] -> BusCreator183/156  "out_pt_ThermoMgt_Stat_PT"
  [L340] -> BusCreator183/157  "out_pt_TotalVehDist_Cval_DIAG"
  [L341] -> BusCreator183/158  "out_pt_TrlrDet_Stat"
  [L342] -> BusCreator183/159  "out_pt_TrqLim_Cval_CPC"
  [L343] -> BusCreator183/160  "out_pt_VehMtn_Stat_PT"
  [L344] -> BusCreator183/161  "out_pt_VehSpd_Cval_CPC"
  [L345] -> BusCreator183/162  "out_pt_VehSpd_Cval_PT"
  [L346] -> BusCreator183/163  "out_pt_VehWeight_Cval_PT"
  [L347] -> BusCreator183/164  "out_pt_VehWeight_Stat_PT"
  [L348] -> BusCreator183/165  "out_pt_WtrPmp_Rq_PT"
  [L349] -> BusCreator183/166  "out_pt_XBR_Stat_PT"
  [L350] -> BusCreator183/167  "out_pt_XSS_Stat"
  [L351] -> BusCreator183/168  "out_cpc_Ignition"
  [L352] -> BusCreator183/169  "out_cpc_TrqDecIdx"
  [L353] -> BusCreator183/170  "out_cpc_ag_g_EngTargetSpeed"
  [L354] -> BusCreator183/171  "out_cpc_ag_m_FiltTrqRatio"
  [L355] -> BusCreator183/172  "out_cpc_cc_p_CcSecure_LowSwitchOnVehSpd_u8"
  [L357] -> out_cpc_itpm_g_RoadGrad_pct/1
  sfunction/173 -> [L357]
  [L358] -> out_cpc_itpm_g_VehMass_t/1
  sfunction/174 -> [L358]
